simulink model "Simulink_Discreate_Test_Model_V2"  (R2018a)
settings: Solver=ode15s  StartTime=0.0  StopTime=7  FixedStep=0.0001  RelTol=1e-3  EnableMultiTasking=on
libraries: discretizing x6
settings Model: Creator=user  LastModifiedBy=user
settings SolverCC: ConcurrentTasks=on  AutoInsertRateTranBlk=on
settings DataIOCC: SaveFormat=StructureWithTime  SaveState=on  SignalLoggingName=logsOut
settings OptimizationCC: BlockReduction=off  BooleanDataType=off  OptimizeBlockIOStorage=off  BufferReuse=off  GlobalBufferReuse=off  ExpressionFolding=off  LocalBlockOutputs=off  InitFltsAndDblsToZero=on  OptimizeDataStoreBuffers=off  BusAssignmentInplaceUpdate=off
settings DebuggingCC: SaveWithParameterizedLinksMsg=none  UnderspecifiedInitializationDetection=Classic  MergeDetectMultiDrivingBlocksExec=none  CheckExecutionContextPreStartOutputMsg=on  CheckExecutionContextRuntimeOutputMsg=on  SignalResolutionControl=TryResolveAllWithWarning  SFUnexpectedBacktrackingDiag=warning  SFNoUnconditionalDefaultTransitionDiag=warning  SFExecutionAtInitializationDiag=none
settings HardwareCC: ProdBitPerPointer=32  ProdBitPerSizeT=32  ProdBitPerPtrDiffT=32  ProdLargestAtomicFloat=None  ProdWordSize=32  ProdLongLongMode=on  ProdHWDeviceType=Generic->32-bit x86 compatible
settings ModelReferenceCC: PropagateSignalLabelsOutOfModel=off
settings RTWCC: SystemTargetFile=slrt.tlc  TemplateMakefile=slrt_default_tmf  Description=Simulink Real-Time  CodeExecutionProfiling=on  RTWCompilerOptimization=on
settings CodeAppCC: StateflowObjectComments=on
settings SimulinkRealTimeCC: SupportVariableSizeSignals=on  RL32LogTETModifier=off  xPCConcurrentTasks=on
settings ConfigComp: CovMetricSettings=dw  CovHtmlReporting=on  CovSaveCumulativeToWorkspaceVar=on  CovSaveSingleToWorkspaceVar=on  CovExternalEMLEnable=off  CovSFcnEnable=off

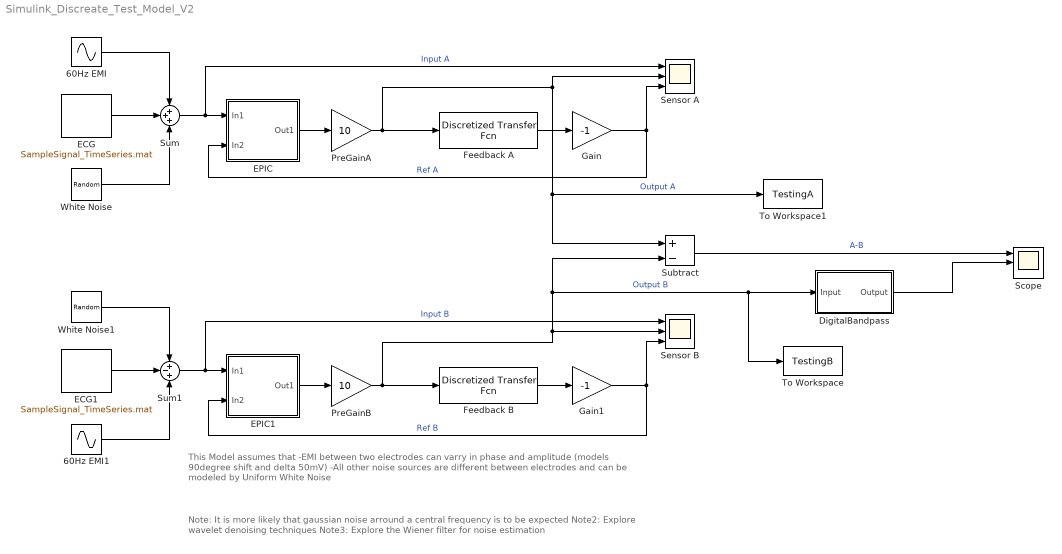
== system Simulink_Discreate_Test_Model_V2 ==
  note: Note: It is more likely that gaussian noise arround a central frequency is to be expected
      | Note2: Explore wavelet denoising techniques
      | Note3: Explore the Wiener filter for noise estimation
  note: This Model assumes that
      | -EMI between two electrodes can varry in phase and amplitude (models 90degree shift and delta 50mV)
      | -All other noise sources are different between electrodes and can be modeled by Uniform White Noise
  60Hz EMI : Sin  Amplitude=0.3  Frequency=377  SampleTime=0.0001
  60Hz EMI1 : Sin  Amplitude=0.35  Frequency=377  Phase=1.97  SampleTime=0.0001
  DigitalBandpass : Subsystem  Tag=FilterWizardSubSystem
      settings: ErrorFcn=dspFilterRealizedInBasicElemsAlgLoopErrFcnCallback
  ECG : FromFile  FileName=SampleSignal_TimeSeries.mat  SampleTime=0
  ECG1 : FromFile  FileName=SampleSignal_TimeSeries.mat  SampleTime=0
  EPIC : Subsystem
  EPIC1 : Subsystem
  Feedback A : discretizing/Discretized Transfer Fcn  Numerator=[1.09 210 25900 59800]  Denominator=[1 19.9 118000 1530]  AbsTol=auto  SampleTime=0.00001  method=matched  Wc=1
  Feedback B : discretizing/Discretized Transfer Fcn  Numerator=[1.09 210 25900 59800]  Denominator=[1 19.9 118000 1530]  AbsTol=auto  SampleTime=0.00001  method=matched  Wc=1
  Gain : Gain  Gain=-1  SaturateOnIntegerOverflow=on  OutDataTypeStr=Inherit: Same as input  ParamDataTypeStr=Inherit: Same as input
  Gain1 : Gain  Gain=-1  SaturateOnIntegerOverflow=on  OutDataTypeStr=Inherit: Same as input  ParamDataTypeStr=Inherit: Same as input
  PreGainA : Gain  Gain=10  OutMin=-5  OutMax=5  SaturateOnIntegerOverflow=on  OutDataTypeStr=Inherit: Same as input  ParamDataTypeStr=Inherit: Same as input
  PreGainB : Gain  Gain=10  OutMin=-5  OutMax=5  SaturateOnIntegerOverflow=on  OutDataTypeStr=Inherit: Same as input  ParamDataTypeStr=Inherit: Same as input
  Scope : Scope  NumInputPorts=3
  Sensor A : Scope  NumInputPorts=3
  Sensor B : Scope  NumInputPorts=3
  Subtract : Sum  Inputs=+-
  Sum : Sum  Inputs=+++
  Sum1 : Sum  Inputs=+-+
  To Workspace : ToWorkspace  VariableName=TestingB  SaveFormat=Timeseries  SampleTime=-1
  To Workspace1 : ToWorkspace  VariableName=TestingA  SaveFormat=Timeseries  SampleTime=-1
  White Noise : UniformRandomNumber  Minimum=-0.1  Maximum=0.1  Seed=523589  SampleTime=0.0001
  White Noise1 : UniformRandomNumber  Minimum=-0.1  Maximum=0.1  SampleTime=0.0001
  wires:
  Gain/1 -> Sensor A/3, EPIC/2(In2)  "Ref A"
  EPIC/1(Out1) -> PreGainA/1
  Feedback A/1 -> Gain/1
  ECG/1 -> Sum/2
  PreGainA/1 -> Feedback A/1, To Workspace1/1, Subtract/1, Sensor A/2  "Output A"
  Sum/1 -> Sensor A/1, EPIC/1(In1)  "Input A"
  Sum1/1 -> Sensor B/1, EPIC1/1(In1)  "Input B"
  PreGainB/1 -> Feedback B/1, Sensor B/2, To Workspace/1, DigitalBandpass/1(Input), Subtract/2  "Output B"
  EPIC1/1(Out1) -> PreGainB/1
  Feedback B/1 -> Gain1/1
  Gain1/1 -> Sensor B/3, EPIC1/2(In2)  "Ref B"
  60Hz EMI/1 -> Sum/1
  60Hz EMI1/1 -> Sum1/3
  ECG1/1 -> Sum1/2
  White Noise/1 -> Sum/3
  Subtract/1 -> Scope/1  "A-B"
  White Noise1/1 -> Sum1/1
  DigitalBandpass/1(Output) -> Scope/2

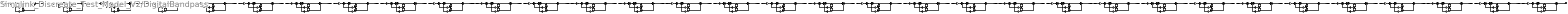
== system Simulink_Discreate_Test_Model_V2/DigitalBandpass ==
  Input : Inport
  Delay{11..19,21..29,110..133,210..233} (66 alike) : Delay  DelayLength=1  InitialCondition=0
  SumA{21..29,31..39,210..233,310..333} (66 alike) : Sum  Inputs=|+-  RndMeth=Nearest  SaturateOnIntegerOverflow=on  OutDataTypeStr=Inherit: Same as first input
  SumB{31..39,310..333} (33 alike) : Sum  Inputs=|+-  RndMeth=Nearest  SaturateOnIntegerOverflow=on  OutDataTypeStr=Inherit: Same as first input
  a(2)(1) : Gain  Gain=-1.94662160591710576  ParamDataTypeStr=double  RndMeth=Nearest  SaturateOnIntegerOverflow=on  OutDataTypeStr=Inherit: Same as input
  a(2)(10) : Gain  Gain=-1.99507563765632945  ParamDataTypeStr=double  RndMeth=Nearest  SaturateOnIntegerOverflow=on  OutDataTypeStr=Inherit: Same as input
  a(2)(11) : Gain  Gain=-1.99402999161732741  ParamDataTypeStr=double  RndMeth=Nearest  SaturateOnIntegerOverflow=on  OutDataTypeStr=Inherit: Same as input
  a(2)(12) : Gain  Gain=-1.80290649306038642  ParamDataTypeStr=double  RndMeth=Nearest  SaturateOnIntegerOverflow=on  OutDataTypeStr=Inherit: Same as input
  a(2)(13) : Gain  Gain=-1.99301133689679233  ParamDataTypeStr=double  RndMeth=Nearest  SaturateOnIntegerOverflow=on  OutDataTypeStr=Inherit: Same as input
  a(2)(14) : Gain  Gain=-1.77988776561854478  ParamDataTypeStr=double  RndMeth=Nearest  SaturateOnIntegerOverflow=on  OutDataTypeStr=Inherit: Same as input
  a(2)(15) : Gain  Gain=-1.99202771048083949  ParamDataTypeStr=double  RndMeth=Nearest  SaturateOnIntegerOverflow=on  OutDataTypeStr=Inherit: Same as input
  a(2)(16) : Gain  Gain=-1.75898489700726035  ParamDataTypeStr=double  RndMeth=Nearest  SaturateOnIntegerOverflow=on  OutDataTypeStr=Inherit: Same as input
  a(2)(17) : Gain  Gain=-1.99108882290856792  ParamDataTypeStr=double  RndMeth=Nearest  SaturateOnIntegerOverflow=on  OutDataTypeStr=Inherit: Same as input
  a(2)(18) : Gain  Gain=-1.74024460415290072  ParamDataTypeStr=double  RndMeth=Nearest  SaturateOnIntegerOverflow=on  OutDataTypeStr=Inherit: Same as input
  a(2)(19) : Gain  Gain=-1.99020622534198743  ParamDataTypeStr=double  RndMeth=Nearest  SaturateOnIntegerOverflow=on  OutDataTypeStr=Inherit: Same as input
  a(2)(2) : Gain  Gain=-1.99941181292600367  ParamDataTypeStr=double  RndMeth=Nearest  SaturateOnIntegerOverflow=on  OutDataTypeStr=Inherit: Same as input
  a(2)(20) : Gain  Gain=-1.72369787635082083  ParamDataTypeStr=double  RndMeth=Nearest  SaturateOnIntegerOverflow=on  OutDataTypeStr=Inherit: Same as input
  a(2)(21) : Gain  Gain=-1.98939333477088276  ParamDataTypeStr=double  RndMeth=Nearest  SaturateOnIntegerOverflow=on  OutDataTypeStr=Inherit: Same as input
  a(2)(22) : Gain  Gain=-1.70936266462510456  ParamDataTypeStr=double  RndMeth=Nearest  SaturateOnIntegerOverflow=on  OutDataTypeStr=Inherit: Same as input
  a(2)(23) : Gain  Gain=-1.98866522847669014  ParamDataTypeStr=double  RndMeth=Nearest  SaturateOnIntegerOverflow=on  OutDataTypeStr=Inherit: Same as input
  a(2)(24) : Gain  Gain=-1.69724645660660345  ParamDataTypeStr=double  RndMeth=Nearest  SaturateOnIntegerOverflow=on  OutDataTypeStr=Inherit: Same as input
  a(2)(25) : Gain  Gain=-1.98803811152960375  ParamDataTypeStr=double  RndMeth=Nearest  SaturateOnIntegerOverflow=on  OutDataTypeStr=Inherit: Same as input
  a(2)(26) : Gain  Gain=-1.68734883145061021  ParamDataTypeStr=double  RndMeth=Nearest  SaturateOnIntegerOverflow=on  OutDataTypeStr=Inherit: Same as input
  a(2)(27) : Gain  Gain=-1.9875283865185609  ParamDataTypeStr=double  RndMeth=Nearest  SaturateOnIntegerOverflow=on  OutDataTypeStr=Inherit: Same as input
  a(2)(28) : Gain  Gain=-1.67966407211069524  ParamDataTypeStr=double  RndMeth=Nearest  SaturateOnIntegerOverflow=on  OutDataTypeStr=Inherit: Same as input
  a(2)(29) : Gain  Gain=-1.9871513315106375  ParamDataTypeStr=double  RndMeth=Nearest  SaturateOnIntegerOverflow=on  OutDataTypeStr=Inherit: Same as input
  a(2)(3) : Gain  Gain=-1.91448793893333002  ParamDataTypeStr=double  RndMeth=Nearest  SaturateOnIntegerOverflow=on  OutDataTypeStr=Inherit: Same as input
  a(2)(30) : Gain  Gain=-1.67418383990444086  ParamDataTypeStr=double  RndMeth=Nearest  SaturateOnIntegerOverflow=on  OutDataTypeStr=Inherit: Same as input
  a(2)(31) : Gain  Gain=-1.98691952202426592  ParamDataTypeStr=double  RndMeth=Nearest  SaturateOnIntegerOverflow=on  OutDataTypeStr=Inherit: Same as input
  a(2)(32) : Gain  Gain=-1.67089978798864114  ParamDataTypeStr=double  RndMeth=Nearest  SaturateOnIntegerOverflow=on  OutDataTypeStr=Inherit: Same as input
  a(2)(33) : Gain  Gain=-1.82832356121550155  ParamDataTypeStr=double  RndMeth=Nearest  SaturateOnIntegerOverflow=on  OutDataTypeStr=Inherit: Same as input
  a(2)(4) : Gain  Gain=-1.99831400657383029  ParamDataTypeStr=double  RndMeth=Nearest  SaturateOnIntegerOverflow=on  OutDataTypeStr=Inherit: Same as input
  a(2)(5) : Gain  Gain=-1.88389275965310032  ParamDataTypeStr=double  RndMeth=Nearest  SaturateOnIntegerOverflow=on  OutDataTypeStr=Inherit: Same as input
  a(2)(6) : Gain  Gain=-1.99722264578434028  ParamDataTypeStr=double  RndMeth=Nearest  SaturateOnIntegerOverflow=on  OutDataTypeStr=Inherit: Same as input
  a(2)(7) : Gain  Gain=-1.85500852743785272  ParamDataTypeStr=double  RndMeth=Nearest  SaturateOnIntegerOverflow=on  OutDataTypeStr=Inherit: Same as input
  a(2)(8) : Gain  Gain=-1.99614167024299682  ParamDataTypeStr=double  RndMeth=Nearest  SaturateOnIntegerOverflow=on  OutDataTypeStr=Inherit: Same as input
  a(2)(9) : Gain  Gain=-1.82797575673544888  ParamDataTypeStr=double  RndMeth=Nearest  SaturateOnIntegerOverflow=on  OutDataTypeStr=Inherit: Same as input
  a(3)(1) : Gain  Gain=0.983099508916992493  ParamDataTypeStr=double  RndMeth=Nearest  SaturateOnIntegerOverflow=on  OutDataTypeStr=Inherit: Same as input
  a(3)(10) : Gain  Gain=0.995114303561969948  ParamDataTypeStr=double  RndMeth=Nearest  SaturateOnIntegerOverflow=on  OutDataTypeStr=Inherit: Same as input
  a(3)(11) : Gain  Gain=0.994069001166917543  ParamDataTypeStr=double  RndMeth=Nearest  SaturateOnIntegerOverflow=on  OutDataTypeStr=Inherit: Same as input
  a(3)(12) : Gain  Gain=0.835712514789545224  ParamDataTypeStr=double  RndMeth=Nearest  SaturateOnIntegerOverflow=on  OutDataTypeStr=Inherit: Same as input
  a(3)(13) : Gain  Gain=0.993050749085394591  ParamDataTypeStr=double  RndMeth=Nearest  SaturateOnIntegerOverflow=on  OutDataTypeStr=Inherit: Same as input
  a(3)(14) : Gain  Gain=0.811924565911670171  ParamDataTypeStr=double  RndMeth=Nearest  SaturateOnIntegerOverflow=on  OutDataTypeStr=Inherit: Same as input
  a(3)(15) : Gain  Gain=0.992067575115055389  ParamDataTypeStr=double  RndMeth=Nearest  SaturateOnIntegerOverflow=on  OutDataTypeStr=Inherit: Same as input
  a(3)(16) : Gain  Gain=0.79026734919360353  ParamDataTypeStr=double  RndMeth=Nearest  SaturateOnIntegerOverflow=on  OutDataTypeStr=Inherit: Same as input
  a(3)(17) : Gain  Gain=0.991129177825510799  ParamDataTypeStr=double  RndMeth=Nearest  SaturateOnIntegerOverflow=on  OutDataTypeStr=Inherit: Same as input
  a(3)(18) : Gain  Gain=0.770799928719128502  ParamDataTypeStr=double  RndMeth=Nearest  SaturateOnIntegerOverflow=on  OutDataTypeStr=Inherit: Same as input
  a(3)(19) : Gain  Gain=0.99024709324345217  ParamDataTypeStr=double  RndMeth=Nearest  SaturateOnIntegerOverflow=on  OutDataTypeStr=Inherit: Same as input
  a(3)(2) : Gain  Gain=0.999449804757627347  ParamDataTypeStr=double  RndMeth=Nearest  SaturateOnIntegerOverflow=on  OutDataTypeStr=Inherit: Same as input
  a(3)(20) : Gain  Gain=0.753566131502359515  ParamDataTypeStr=double  RndMeth=Nearest  SaturateOnIntegerOverflow=on  OutDataTypeStr=Inherit: Same as input
  a(3)(21) : Gain  Gain=0.989434719859647149  ParamDataTypeStr=double  RndMeth=Nearest  SaturateOnIntegerOverflow=on  OutDataTypeStr=Inherit: Same as input
  a(3)(22) : Gain  Gain=0.738597150892476906  ParamDataTypeStr=double  RndMeth=Nearest  SaturateOnIntegerOverflow=on  OutDataTypeStr=Inherit: Same as input
  a(3)(23) : Gain  Gain=0.988707113256216519  ParamDataTypeStr=double  RndMeth=Nearest  SaturateOnIntegerOverflow=on  OutDataTypeStr=Inherit: Same as input
  a(3)(24) : Gain  Gain=0.725913919094523963  ParamDataTypeStr=double  RndMeth=Nearest  SaturateOnIntegerOverflow=on  OutDataTypeStr=Inherit: Same as input
  a(3)(25) : Gain  Gain=0.988080454327139535  ParamDataTypeStr=double  RndMeth=Nearest  SaturateOnIntegerOverflow=on  OutDataTypeStr=Inherit: Same as input
  a(3)(26) : Gain  Gain=0.715529297111775375  ParamDataTypeStr=double  RndMeth=Nearest  SaturateOnIntegerOverflow=on  OutDataTypeStr=Inherit: Same as input
  a(3)(27) : Gain  Gain=0.987571120455381757  ParamDataTypeStr=double  RndMeth=Nearest  SaturateOnIntegerOverflow=on  OutDataTypeStr=Inherit: Same as input
  a(3)(28) : Gain  Gain=0.707450129651092996  ParamDataTypeStr=double  RndMeth=Nearest  SaturateOnIntegerOverflow=on  OutDataTypeStr=Inherit: Same as input
  a(3)(29) : Gain  Gain=0.987194365671987484  ParamDataTypeStr=double  RndMeth=Nearest  SaturateOnIntegerOverflow=on  OutDataTypeStr=Inherit: Same as input
  a(3)(3) : Gain  Gain=0.950290088498272012  ParamDataTypeStr=double  RndMeth=Nearest  SaturateOnIntegerOverflow=on  OutDataTypeStr=Inherit: Same as input
  a(3)(30) : Gain  Gain=0.701679180433258609  ParamDataTypeStr=double  RndMeth=Nearest  SaturateOnIntegerOverflow=on  OutDataTypeStr=Inherit: Same as input
  a(3)(31) : Gain  Gain=0.986962745359862281  ParamDataTypeStr=double  RndMeth=Nearest  SaturateOnIntegerOverflow=on  OutDataTypeStr=Inherit: Same as input
  a(3)(32) : Gain  Gain=0.698216898573133515  ParamDataTypeStr=double  RndMeth=Nearest  SaturateOnIntegerOverflow=on  OutDataTypeStr=Inherit: Same as input
  a(3)(33) : Gain  Gain=0.829409794328705763  ParamDataTypeStr=double  RndMeth=Nearest  SaturateOnIntegerOverflow=on  OutDataTypeStr=Inherit: Same as input
  a(3)(4) : Gain  Gain=0.998352054878109629  ParamDataTypeStr=double  RndMeth=Nearest  SaturateOnIntegerOverflow=on  OutDataTypeStr=Inherit: Same as input
  a(3)(5) : Gain  Gain=0.918979727798706403  ParamDataTypeStr=double  RndMeth=Nearest  SaturateOnIntegerOverflow=on  OutDataTypeStr=Inherit: Same as input
  a(3)(6) : Gain  Gain=0.997260826893489272  ParamDataTypeStr=double  RndMeth=Nearest  SaturateOnIntegerOverflow=on  OutDataTypeStr=Inherit: Same as input
  a(3)(7) : Gain  Gain=0.889350742457201027  ParamDataTypeStr=double  RndMeth=Nearest  SaturateOnIntegerOverflow=on  OutDataTypeStr=Inherit: Same as input
  a(3)(8) : Gain  Gain=0.996180058353088538  ParamDataTypeStr=double  RndMeth=Nearest  SaturateOnIntegerOverflow=on  OutDataTypeStr=Inherit: Same as input
  a(3)(9) : Gain  Gain=0.861554032761983279  ParamDataTypeStr=double  RndMeth=Nearest  SaturateOnIntegerOverflow=on  OutDataTypeStr=Inherit: Same as input
  s(1) : Gain  Gain=0.0924402491442333357  ParamDataTypeStr=double  RndMeth=Nearest  SaturateOnIntegerOverflow=on  OutDataTypeStr=Inherit: Same as input
  s(10) : Gain  Gain=0.0894734842322397333  ParamDataTypeStr=double  RndMeth=Nearest  SaturateOnIntegerOverflow=on  OutDataTypeStr=Inherit: Same as input
  s(11) : Gain  Gain=0.0888307463997321939  ParamDataTypeStr=double  RndMeth=Nearest  SaturateOnIntegerOverflow=on  OutDataTypeStr=Inherit: Same as input
  s(12) : Gain  Gain=0.0888307463997321939  ParamDataTypeStr=double  RndMeth=Nearest  SaturateOnIntegerOverflow=on  OutDataTypeStr=Inherit: Same as input
  s(13) : Gain  Gain=0.0882350025183955416  ParamDataTypeStr=double  RndMeth=Nearest  SaturateOnIntegerOverflow=on  OutDataTypeStr=Inherit: Same as input
  s(14) : Gain  Gain=0.0882350025183955416  ParamDataTypeStr=double  RndMeth=Nearest  SaturateOnIntegerOverflow=on  OutDataTypeStr=Inherit: Same as input
  s(15) : Gain  Gain=0.0876890460826875578  ParamDataTypeStr=double  RndMeth=Nearest  SaturateOnIntegerOverflow=on  OutDataTypeStr=Inherit: Same as input
  s(16) : Gain  Gain=0.0876890460826875578  ParamDataTypeStr=double  RndMeth=Nearest  SaturateOnIntegerOverflow=on  OutDataTypeStr=Inherit: Same as input
  s(17) : Gain  Gain=0.0871952322840942318  ParamDataTypeStr=double  RndMeth=Nearest  SaturateOnIntegerOverflow=on  OutDataTypeStr=Inherit: Same as input
  s(18) : Gain  Gain=0.0871952322840942318  ParamDataTypeStr=double  RndMeth=Nearest  SaturateOnIntegerOverflow=on  OutDataTypeStr=Inherit: Same as input
  s(19) : Gain  Gain=0.0867555274599517423  ParamDataTypeStr=double  RndMeth=Nearest  SaturateOnIntegerOverflow=on  OutDataTypeStr=Inherit: Same as input
  s(2) : Gain  Gain=0.0924402491442333357  ParamDataTypeStr=double  RndMeth=Nearest  SaturateOnIntegerOverflow=on  OutDataTypeStr=Inherit: Same as input
  s(20) : Gain  Gain=0.0867555274599517423  ParamDataTypeStr=double  RndMeth=Nearest  SaturateOnIntegerOverflow=on  OutDataTypeStr=Inherit: Same as input
  s(21) : Gain  Gain=0.0863715548885271717  ParamDataTypeStr=double  RndMeth=Nearest  SaturateOnIntegerOverflow=on  OutDataTypeStr=Inherit: Same as input
  s(22) : Gain  Gain=0.0863715548885271717  ParamDataTypeStr=double  RndMeth=Nearest  SaturateOnIntegerOverflow=on  OutDataTypeStr=Inherit: Same as input
  s(23) : Gain  Gain=0.0860446361148538424  ParamDataTypeStr=double  RndMeth=Nearest  SaturateOnIntegerOverflow=on  OutDataTypeStr=Inherit: Same as input
  s(24) : Gain  Gain=0.0860446361148538424  ParamDataTypeStr=double  RndMeth=Nearest  SaturateOnIntegerOverflow=on  OutDataTypeStr=Inherit: Same as input
  s(25) : Gain  Gain=0.0857758272667807353  ParamDataTypeStr=double  RndMeth=Nearest  SaturateOnIntegerOverflow=on  OutDataTypeStr=Inherit: Same as input
  s(26) : Gain  Gain=0.0857758272667807353  ParamDataTypeStr=double  RndMeth=Nearest  SaturateOnIntegerOverflow=on  OutDataTypeStr=Inherit: Same as input
  s(27) : Gain  Gain=0.0855659500261026218  ParamDataTypeStr=double  RndMeth=Nearest  SaturateOnIntegerOverflow=on  OutDataTypeStr=Inherit: Same as input
  s(28) : Gain  Gain=0.0855659500261026218  ParamDataTypeStr=double  RndMeth=Nearest  SaturateOnIntegerOverflow=on  OutDataTypeStr=Inherit: Same as input
  s(29) : Gain  Gain=0.0854156170655830382  ParamDataTypeStr=double  RndMeth=Nearest  SaturateOnIntegerOverflow=on  OutDataTypeStr=Inherit: Same as input
  s(3) : Gain  Gain=0.0916480572815368266  ParamDataTypeStr=double  RndMeth=Nearest  SaturateOnIntegerOverflow=on  OutDataTypeStr=Inherit: Same as input
  s(30) : Gain  Gain=0.0854156170655830382  ParamDataTypeStr=double  RndMeth=Nearest  SaturateOnIntegerOverflow=on  OutDataTypeStr=Inherit: Same as input
  s(31) : Gain  Gain=0.0853252518597319293  ParamDataTypeStr=double  RndMeth=Nearest  SaturateOnIntegerOverflow=on  OutDataTypeStr=Inherit: Same as input
  s(32) : Gain  Gain=0.0853252518597319293  ParamDataTypeStr=double  RndMeth=Nearest  SaturateOnIntegerOverflow=on  OutDataTypeStr=Inherit: Same as input
  s(33) : Gain  Gain=0.085295102835647188  ParamDataTypeStr=double  RndMeth=Nearest  SaturateOnIntegerOverflow=on  OutDataTypeStr=Inherit: Same as input
  s(4) : Gain  Gain=0.0916480572815368266  ParamDataTypeStr=double  RndMeth=Nearest  SaturateOnIntegerOverflow=on  OutDataTypeStr=Inherit: Same as input
  s(5) : Gain  Gain=0.0908862637717108846  ParamDataTypeStr=double  RndMeth=Nearest  SaturateOnIntegerOverflow=on  OutDataTypeStr=Inherit: Same as input
  s(6) : Gain  Gain=0.0908862637717108846  ParamDataTypeStr=double  RndMeth=Nearest  SaturateOnIntegerOverflow=on  OutDataTypeStr=Inherit: Same as input
  s(7) : Gain  Gain=0.0901599322843195244  ParamDataTypeStr=double  RndMeth=Nearest  SaturateOnIntegerOverflow=on  OutDataTypeStr=Inherit: Same as input
  s(8) : Gain  Gain=0.0901599322843195244  ParamDataTypeStr=double  RndMeth=Nearest  SaturateOnIntegerOverflow=on  OutDataTypeStr=Inherit: Same as input
  s(9) : Gain  Gain=0.0894734842322397333  ParamDataTypeStr=double  RndMeth=Nearest  SaturateOnIntegerOverflow=on  OutDataTypeStr=Inherit: Same as input
  Output : Outport
  wires:
  Input/1 -> s(1)/1
  s(1)/1 -> SumA21/1
  SumA21/1 -> SumA31/1
  SumA31/1 -> SumB31/1, Delay11/1
  SumB31/1 -> [Sect1]
  a(2)(1)/1 -> SumA21/2
  Delay11/1 -> a(2)(1)/1, Delay21/1
  a(3)(1)/1 -> SumA31/2
  Delay21/1 -> a(3)(1)/1, SumB31/2
  [Sect1] -> s(2)/1
  s(2)/1 -> SumA22/1
  SumA22/1 -> SumA32/1
  SumA32/1 -> SumB32/1, Delay12/1
  SumB32/1 -> [Sect2]
  a(2)(2)/1 -> SumA22/2
  Delay12/1 -> a(2)(2)/1, Delay22/1
  a(3)(2)/1 -> SumA32/2
  Delay22/1 -> a(3)(2)/1, SumB32/2
  [Sect2] -> s(3)/1
  s(3)/1 -> SumA23/1
  SumA23/1 -> SumA33/1
  SumA33/1 -> SumB33/1, Delay13/1
  SumB33/1 -> [Sect3]
  a(2)(3)/1 -> SumA23/2
  Delay13/1 -> a(2)(3)/1, Delay23/1
  a(3)(3)/1 -> SumA33/2
  Delay23/1 -> a(3)(3)/1, SumB33/2
  [Sect3] -> s(4)/1
  s(4)/1 -> SumA24/1
  SumA24/1 -> SumA34/1
  SumA34/1 -> SumB34/1, Delay14/1
  SumB34/1 -> [Sect4]
  a(2)(4)/1 -> SumA24/2
  Delay14/1 -> a(2)(4)/1, Delay24/1
  a(3)(4)/1 -> SumA34/2
  Delay24/1 -> a(3)(4)/1, SumB34/2
  [Sect4] -> s(5)/1
  s(5)/1 -> SumA25/1
  SumA25/1 -> SumA35/1
  SumA35/1 -> SumB35/1, Delay15/1
  SumB35/1 -> [Sect5]
  a(2)(5)/1 -> SumA25/2
  Delay15/1 -> a(2)(5)/1, Delay25/1
  a(3)(5)/1 -> SumA35/2
  Delay25/1 -> a(3)(5)/1, SumB35/2
  [Sect5] -> s(6)/1
  s(6)/1 -> SumA26/1
  SumA26/1 -> SumA36/1
  SumA36/1 -> SumB36/1, Delay16/1
  SumB36/1 -> [Sect6]
  a(2)(6)/1 -> SumA26/2
  Delay16/1 -> a(2)(6)/1, Delay26/1
  a(3)(6)/1 -> SumA36/2
  Delay26/1 -> a(3)(6)/1, SumB36/2
  [Sect6] -> s(7)/1
  s(7)/1 -> SumA27/1
  SumA27/1 -> SumA37/1
  SumA37/1 -> SumB37/1, Delay17/1
  SumB37/1 -> [Sect7]
  a(2)(7)/1 -> SumA27/2
  Delay17/1 -> a(2)(7)/1, Delay27/1
  a(3)(7)/1 -> SumA37/2
  Delay27/1 -> a(3)(7)/1, SumB37/2
  [Sect7] -> s(8)/1
  s(8)/1 -> SumA28/1
  SumA28/1 -> SumA38/1
  SumA38/1 -> SumB38/1, Delay18/1
  SumB38/1 -> [Sect8]
  a(2)(8)/1 -> SumA28/2
  Delay18/1 -> a(2)(8)/1, Delay28/1
  a(3)(8)/1 -> SumA38/2
  Delay28/1 -> a(3)(8)/1, SumB38/2
  [Sect8] -> s(9)/1
  s(9)/1 -> SumA29/1
  SumA29/1 -> SumA39/1
  SumA39/1 -> SumB39/1, Delay19/1
  SumB39/1 -> [Sect9]
  a(2)(9)/1 -> SumA29/2
  Delay19/1 -> a(2)(9)/1, Delay29/1
  a(3)(9)/1 -> SumA39/2
  Delay29/1 -> a(3)(9)/1, SumB39/2
  [Sect9] -> s(10)/1
  s(10)/1 -> SumA210/1
  SumA210/1 -> SumA310/1
  SumA310/1 -> SumB310/1, Delay110/1
  SumB310/1 -> [Sect10]
  a(2)(10)/1 -> SumA210/2
  Delay110/1 -> a(2)(10)/1, Delay210/1
  a(3)(10)/1 -> SumA310/2
  Delay210/1 -> a(3)(10)/1, SumB310/2
  [Sect10] -> s(11)/1
  s(11)/1 -> SumA211/1
  SumA211/1 -> SumA311/1
  SumA311/1 -> SumB311/1, Delay111/1
  SumB311/1 -> [Sect11]
  a(2)(11)/1 -> SumA211/2
  Delay111/1 -> a(2)(11)/1, Delay211/1
  a(3)(11)/1 -> SumA311/2
  Delay211/1 -> a(3)(11)/1, SumB311/2
  [Sect11] -> s(12)/1
  s(12)/1 -> SumA212/1
  SumA212/1 -> SumA312/1
  SumA312/1 -> SumB312/1, Delay112/1
  SumB312/1 -> [Sect12]
  a(2)(12)/1 -> SumA212/2
  Delay112/1 -> a(2)(12)/1, Delay212/1
  a(3)(12)/1 -> SumA312/2
  Delay212/1 -> a(3)(12)/1, SumB312/2
  [Sect12] -> s(13)/1
  s(13)/1 -> SumA213/1
  SumA213/1 -> SumA313/1
  SumA313/1 -> SumB313/1, Delay113/1
  SumB313/1 -> [Sect13]
  a(2)(13)/1 -> SumA213/2
  Delay113/1 -> a(2)(13)/1, Delay213/1
  a(3)(13)/1 -> SumA313/2
  Delay213/1 -> a(3)(13)/1, SumB313/2
  [Sect13] -> s(14)/1
  s(14)/1 -> SumA214/1
  SumA214/1 -> SumA314/1
  SumA314/1 -> SumB314/1, Delay114/1
  SumB314/1 -> [Sect14]
  a(2)(14)/1 -> SumA214/2
  Delay114/1 -> a(2)(14)/1, Delay214/1
  a(3)(14)/1 -> SumA314/2
  Delay214/1 -> a(3)(14)/1, SumB314/2
  [Sect14] -> s(15)/1
  s(15)/1 -> SumA215/1
  SumA215/1 -> SumA315/1
  SumA315/1 -> SumB315/1, Delay115/1
  SumB315/1 -> [Sect15]
  a(2)(15)/1 -> SumA215/2
  Delay115/1 -> a(2)(15)/1, Delay215/1
  a(3)(15)/1 -> SumA315/2
  Delay215/1 -> a(3)(15)/1, SumB315/2
  [Sect15] -> s(16)/1
  s(16)/1 -> SumA216/1
  SumA216/1 -> SumA316/1
  SumA316/1 -> SumB316/1, Delay116/1
  SumB316/1 -> [Sect16]
  a(2)(16)/1 -> SumA216/2
  Delay116/1 -> a(2)(16)/1, Delay216/1
  a(3)(16)/1 -> SumA316/2
  Delay216/1 -> a(3)(16)/1, SumB316/2
  [Sect16] -> s(17)/1
  s(17)/1 -> SumA217/1
  SumA217/1 -> SumA317/1
  SumA317/1 -> SumB317/1, Delay117/1
  SumB317/1 -> [Sect17]
  a(2)(17)/1 -> SumA217/2
  Delay117/1 -> a(2)(17)/1, Delay217/1
  a(3)(17)/1 -> SumA317/2
  Delay217/1 -> a(3)(17)/1, SumB317/2
  [Sect17] -> s(18)/1
  s(18)/1 -> SumA218/1
  SumA218/1 -> SumA318/1
  SumA318/1 -> SumB318/1, Delay118/1
  SumB318/1 -> [Sect18]
  a(2)(18)/1 -> SumA218/2
  Delay118/1 -> a(2)(18)/1, Delay218/1
  a(3)(18)/1 -> SumA318/2
  Delay218/1 -> a(3)(18)/1, SumB318/2
  [Sect18] -> s(19)/1
  s(19)/1 -> SumA219/1
  SumA219/1 -> SumA319/1
  SumA319/1 -> SumB319/1, Delay119/1
  SumB319/1 -> [Sect19]
  a(2)(19)/1 -> SumA219/2
  Delay119/1 -> a(2)(19)/1, Delay219/1
  a(3)(19)/1 -> SumA319/2
  Delay219/1 -> a(3)(19)/1, SumB319/2
  [Sect19] -> s(20)/1
  s(20)/1 -> SumA220/1
  SumA220/1 -> SumA320/1
  SumA320/1 -> SumB320/1, Delay120/1
  SumB320/1 -> [Sect20]
  a(2)(20)/1 -> SumA220/2
  Delay120/1 -> a(2)(20)/1, Delay220/1
  a(3)(20)/1 -> SumA320/2
  Delay220/1 -> a(3)(20)/1, SumB320/2
  [Sect20] -> s(21)/1
  s(21)/1 -> SumA221/1
  SumA221/1 -> SumA321/1
  SumA321/1 -> SumB321/1, Delay121/1
  SumB321/1 -> [Sect21]
  a(2)(21)/1 -> SumA221/2
  Delay121/1 -> a(2)(21)/1, Delay221/1
  a(3)(21)/1 -> SumA321/2
  Delay221/1 -> a(3)(21)/1, SumB321/2
  [Sect21] -> s(22)/1
  s(22)/1 -> SumA222/1
  SumA222/1 -> SumA322/1
  SumA322/1 -> SumB322/1, Delay122/1
  SumB322/1 -> [Sect22]
  a(2)(22)/1 -> SumA222/2
  Delay122/1 -> a(2)(22)/1, Delay222/1
  a(3)(22)/1 -> SumA322/2
  Delay222/1 -> a(3)(22)/1, SumB322/2
  [Sect22] -> s(23)/1
  s(23)/1 -> SumA223/1
  SumA223/1 -> SumA323/1
  SumA323/1 -> SumB323/1, Delay123/1
  SumB323/1 -> [Sect23]
  a(2)(23)/1 -> SumA223/2
  Delay123/1 -> a(2)(23)/1, Delay223/1
  a(3)(23)/1 -> SumA323/2
  Delay223/1 -> a(3)(23)/1, SumB323/2
  [Sect23] -> s(24)/1
  s(24)/1 -> SumA224/1
  SumA224/1 -> SumA324/1
  SumA324/1 -> SumB324/1, Delay124/1
  SumB324/1 -> [Sect24]
  a(2)(24)/1 -> SumA224/2
  Delay124/1 -> a(2)(24)/1, Delay224/1
  a(3)(24)/1 -> SumA324/2
  Delay224/1 -> a(3)(24)/1, SumB324/2
  [Sect24] -> s(25)/1
  s(25)/1 -> SumA225/1
  SumA225/1 -> SumA325/1
  SumA325/1 -> SumB325/1, Delay125/1
  SumB325/1 -> [Sect25]
  a(2)(25)/1 -> SumA225/2
  Delay125/1 -> a(2)(25)/1, Delay225/1
  a(3)(25)/1 -> SumA325/2
  Delay225/1 -> a(3)(25)/1, SumB325/2
  [Sect25] -> s(26)/1
  s(26)/1 -> SumA226/1
  SumA226/1 -> SumA326/1
  SumA326/1 -> SumB326/1, Delay126/1
  SumB326/1 -> [Sect26]
  a(2)(26)/1 -> SumA226/2
  Delay126/1 -> a(2)(26)/1, Delay226/1
  a(3)(26)/1 -> SumA326/2
  Delay226/1 -> a(3)(26)/1, SumB326/2
  [Sect26] -> s(27)/1
  s(27)/1 -> SumA227/1
  SumA227/1 -> SumA327/1
  SumA327/1 -> SumB327/1, Delay127/1
  SumB327/1 -> [Sect27]
  a(2)(27)/1 -> SumA227/2
  Delay127/1 -> a(2)(27)/1, Delay227/1
  a(3)(27)/1 -> SumA327/2
  Delay227/1 -> a(3)(27)/1, SumB327/2
  [Sect27] -> s(28)/1
  s(28)/1 -> SumA228/1
  SumA228/1 -> SumA328/1
  SumA328/1 -> SumB328/1, Delay128/1
  SumB328/1 -> [Sect28]
  a(2)(28)/1 -> SumA228/2
  Delay128/1 -> a(2)(28)/1, Delay228/1
  a(3)(28)/1 -> SumA328/2
  Delay228/1 -> a(3)(28)/1, SumB328/2
  [Sect28] -> s(29)/1
  s(29)/1 -> SumA229/1
  SumA229/1 -> SumA329/1
  SumA329/1 -> SumB329/1, Delay129/1
  SumB329/1 -> [Sect29]
  a(2)(29)/1 -> SumA229/2
  Delay129/1 -> a(2)(29)/1, Delay229/1
  a(3)(29)/1 -> SumA329/2
  Delay229/1 -> a(3)(29)/1, SumB329/2
  [Sect29] -> s(30)/1
  s(30)/1 -> SumA230/1
  SumA230/1 -> SumA330/1
  SumA330/1 -> SumB330/1, Delay130/1
  SumB330/1 -> [Sect30]
  a(2)(30)/1 -> SumA230/2
  Delay130/1 -> a(2)(30)/1, Delay230/1
  a(3)(30)/1 -> SumA330/2
  Delay230/1 -> a(3)(30)/1, SumB330/2
  [Sect30] -> s(31)/1
  s(31)/1 -> SumA231/1
  SumA231/1 -> SumA331/1
  SumA331/1 -> SumB331/1, Delay131/1
  SumB331/1 -> [Sect31]
  a(2)(31)/1 -> SumA231/2
  Delay131/1 -> a(2)(31)/1, Delay231/1
  a(3)(31)/1 -> SumA331/2
  Delay231/1 -> a(3)(31)/1, SumB331/2
  [Sect31] -> s(32)/1
  s(32)/1 -> SumA232/1
  SumA232/1 -> SumA332/1
  SumA332/1 -> SumB332/1, Delay132/1
  SumB332/1 -> [Sect32]
  a(2)(32)/1 -> SumA232/2
  Delay132/1 -> a(2)(32)/1, Delay232/1
  a(3)(32)/1 -> SumA332/2
  Delay232/1 -> a(3)(32)/1, SumB332/2
  [Sect32] -> s(33)/1
  s(33)/1 -> SumA233/1
  SumA233/1 -> SumA333/1
  SumA333/1 -> SumB333/1, Delay133/1
  SumB333/1 -> Output/1
  a(2)(33)/1 -> SumA233/2
  Delay133/1 -> a(2)(33)/1, Delay233/1
  a(3)(33)/1 -> SumA333/2
  Delay233/1 -> a(3)(33)/1, SumB333/2

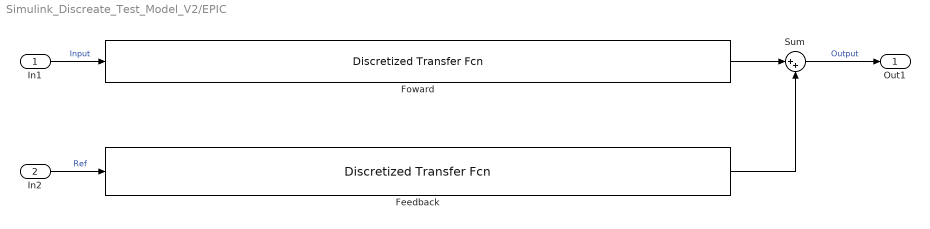
== system Simulink_Discreate_Test_Model_V2/EPIC ==
  In1 : Inport
  In2 : Inport  Port=2
  Feedback : discretizing/Discretized Transfer Fcn  Numerator=[12605.4554063995,23229713663.4924,17234152953470.8,4398216306223.24,3018119162321.11]  Denominator=[1,1423447.52999193,9421519136.03560,6422247005442.77,51913333436888.3,69117764201530.7]  AbsTol=auto  SampleTime=0.00001  method=matched  Wc=1
  Foward : discretizing/Discretized Transfer Fcn  Numerator=[0,0,-40596496340164.1,-10055203430225.6,7778571084474.48]  Denominator=[1,3502079.68268747,5589807862084.53,40022776635817.3,58077323621970.0]  AbsTol=auto  SampleTime=0.00001  method=matched  Wc=1
  Sum : Sum  Inputs=|++  OutMin=[-100]  OutMax=[100]
  Out1 : Outport
  wires:
  In1/1 -> Foward/1  "Input"
  Sum/1 -> Out1/1  "Output"
  In2/1 -> Feedback/1  "Ref"
  Foward/1 -> Sum/1
  Feedback/1 -> Sum/2

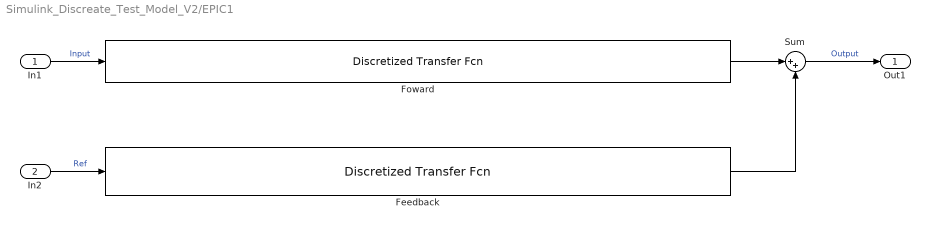
== system Simulink_Discreate_Test_Model_V2/EPIC1 ==
  In1 : Inport
  In2 : Inport  Port=2
  Feedback : discretizing/Discretized Transfer Fcn  Numerator=[12605.4554063995,23229713663.4924,17234152953470.8,4398216306223.24,3018119162321.11]  Denominator=[1,1423447.52999193,9421519136.03560,6422247005442.77,51913333436888.3,69117764201530.7]  AbsTol=auto  SampleTime=0.00001  method=matched  Wc=1
  Foward : discretizing/Discretized Transfer Fcn  Numerator=[0,0,-40596496340164.1,-10055203430225.6,7778571084474.48]  Denominator=[1,3502079.68268747,5589807862084.53,40022776635817.3,58077323621970.0]  AbsTol=auto  SampleTime=0.00001  method=matched  Wc=1
  Sum : Sum  Inputs=|++  OutMin=[-100]  OutMax=[100]
  Out1 : Outport
  wires:
  In1/1 -> Foward/1  "Input"
  Sum/1 -> Out1/1  "Output"
  In2/1 -> Feedback/1  "Ref"
  Foward/1 -> Sum/1
  Feedback/1 -> Sum/2
